simulink model "SS_Model"  (R2019b)
settings: Solver=VariableStepAuto  StartTime=0.0  StopTime=10.0  RelTol=1e-3
model workspace (MATLAB code in the model file):
  | q = 20
  | Cain = 0.8
  | cp = 0.8
  | rho = 52
  | dH = -500
  | Ti = 90
undefined symbols (not defined in the file or in its folder): ca0, T0, V
settings Model: Creator=Raj  LastModifiedBy=Raj

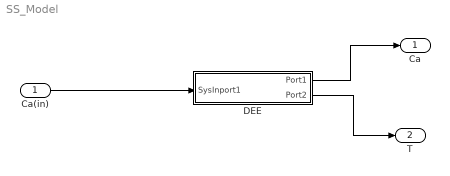
== system SS_Model ==
  Ca(in) : Inport
  DEE : Subsystem  mask(Differential Equation Editor (DEE)){}
      settings: OpenFcn=diffeqed
      mask Display: disp('CSTR')
  Ca : Outport
  T : Outport  Port=2
  wires:
  Ca(in)/1 -> DEE/1(SysInport1)
  DEE/1(Port1) -> Ca/1
  DEE/2(Port2) -> T/1

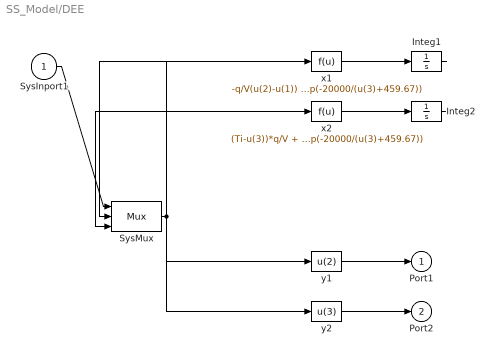
== system SS_Model/DEE ==
  SysInport1 : Inport
  Integ1 : Integrator  InitialCondition=ca0
  Integ2 : Integrator  InitialCondition=T0
  SysMux : Mux  Inputs=3
  x1 : Fcn  Expr=-q/V(u(2)-u(1)) + u(2)*2.4*10^15*exp(-20000/(u(3)+459.67))
  x2 : Fcn  Expr=(Ti-u(3))*q/V + dH/(rho*cp)*u(2)*2.4*10^15*exp(-20000/(u(3)+459.67))
  y1 : Fcn  Expr=u(2)
  y2 : Fcn  Expr=u(3)
  Port1 : Outport
  Port2 : Outport  Port=2
  wires:
  SysInport1/1 -> SysMux/1
  SysMux/1 -> x1/1, x2/1, y1/1, y2/1
  x1/1 -> Integ1/1
  Integ1/1 -> SysMux/2
  x2/1 -> Integ2/1
  Integ2/1 -> SysMux/3
  y1/1 -> Port1/1
  y2/1 -> Port2/1
